simulink model "D53_LKAS_JLU_20200911_1116"  (R2018b)
settings: Solver=ode3  StartTime=0.0  StopTime=10.0  FixedStep=0.01  RelTol=1e-3  EnableMultiTasking=on
model workspace (MAT data in the model file):
  MCOS : class17 (value not decoded)
  MCOS : class17 (value not decoded)
  MCOS : class17 (value not decoded)
  MCOS : class17 (value not decoded)
  MCOS : class17 (value not decoded)
  MCOS : class17 (value not decoded)
  MCOS : class17 (value not decoded)
  MCOS : class17 (value not decoded)
  MCOS : class17 (value not decoded)
  MCOS : class17 (value not decoded)
  MCOS : class17 (value not decoded)
  MCOS : class17 (value not decoded)
  MCOS : class17 (value not decoded)
  MCOS : class17 (value not decoded)
  MCOS : class17 (value not decoded)
  MCOS : class17 (value not decoded)
  MCOS : class17 (value not decoded)
  MCOS : class17 (value not decoded)
  MCOS : class17 (value not decoded)
  MCOS : class17 (value not decoded)
  MCOS : class17 (value not decoded)
  MCOS : class17 (value not decoded)
  MCOS : class17 (value not decoded)
  MCOS : class17 (value not decoded)
  MCOS : class17 (value not decoded)
  MCOS : class17 (value not decoded)
  MCOS : class17 (value not decoded)
  MCOS : class17 (value not decoded)
  MCOS : class17 (value not decoded)
  MCOS : class17 (value not decoded)
  MCOS : class17 (value not decoded)
  MCOS : class17 (value not decoded)
  MCOS : class17 (value not decoded)
  MCOS : class17 (value not decoded)
  MCOS : class17 (value not decoded)
  MCOS : class17 (value not decoded)
  MCOS : class17 (value not decoded)
  MCOS : class17 (value not decoded)
  MCOS : class17 (value not decoded)
  MCOS : class17 (value not decoded)
  MCOS : class17 (value not decoded)
  MCOS : class17 (value not decoded)
  MCOS : class17 (value not decoded)
  MCOS : class17 (value not decoded)
  MCOS : class17 (value not decoded)
  MCOS : class17 (value not decoded)
  MCOS : class17 (value not decoded)
  MCOS : class17 (value not decoded)
  MCOS : class17 (value not decoded)
  MCOS : class17 (value not decoded)
  MCOS : class17 (value not decoded)
  MCOS : class17 (value not decoded)
  MCOS : class17 (value not decoded)
  MCOS : class17 (value not decoded)
  MCOS : class17 (value not decoded)
  MCOS : class17 (value not decoded)
  MCOS : class17 (value not decoded)
  MCOS : class17 (value not decoded)
  MCOS : class17 (value not decoded)
  MCOS : class17 (value not decoded)
  MCOS : class17 (value not decoded)
  MCOS : class17 (value not decoded)
  MCOS : class17 (value not decoded)
  MCOS : class17 (value not decoded)
  MCOS : class17 (value not decoded)
  MCOS : class17 (value not decoded)
  MCOS : class17 (value not decoded)
  MCOS : class17 (value not decoded)
  MCOS : class17 (value not decoded)
  MCOS : class17 (value not decoded)
  MCOS : class17 (value not decoded)
  MCOS : class17 (value not decoded)
  MCOS : class17 (value not decoded)
  MCOS : class17 (value not decoded)
  MCOS : class17 (value not decoded)
  MCOS : class17 (value not decoded)
  MCOS : class17 (value not decoded)
  MCOS : class17 (value not decoded)
  MCOS : class17 (value not decoded)
  MCOS : class17 (value not decoded)
  MCOS : class17 (value not decoded)
  MCOS : class17 (value not decoded)
  MCOS : class17 (value not decoded)
  MCOS : class17 (value not decoded)
  MCOS : class17 (value not decoded)
  MCOS : class17 (value not decoded)
  MCOS : class17 (value not decoded)
  MCOS : class17 (value not decoded)
  MCOS : class17 (value not decoded)
undefined symbols (not defined in the file): LKA_CarWidth, LKA_SampleTime, LKA_StrRatio_C, LKA_Veh2CamL_C, LKA_Veh2CamW_C, LKA_WhlBaseL_C, LL_CompSWA_C, LL_CrvtPrvwT_C, LL_DesDvt_C, LL_DvtComp_C, LL_DvtPrvwT_C, LL_DvtSpdDet_vDvtSpdMin_C, LL_HdAgExT_C, LL_HdAgPrvwT_C, LL_LAccMax_C, LL_LAccRMax_C, LL_LDW_EarliestWarnLine_C, LL_LDW_LatestWarnLine_C, LL_LDWS_SUPPRESS_HEADING, LL_LFClb_TFC_DiffCtlBalance, LL_LFClb_TFC_DiffCtrlMaxSWA, LL_LFClb_TFC_DiffCtrlRatio, LL_LFClb_TFC_facmGainLutGain1_C, LL_LFClb_TFC_facmGainLutGain2_C, LL_LFClb_TFC_facmIntegRatio, LL_LFClb_TFC_facmKlat_C, LL_LFClb_TFC_FfCtlRatio_C, LL_LFClb_TFC_phiIntegCtlMaxSWA_C, LL_LFClb_TFC_tiKlatPrvwT_C, LL_LFClb_TFC_vGainLutVehSpdLwr_C, LL_LFClb_TFC_vGainLutVehSpdUpr_C, LL_LKA_EarliestWarnLine_C, LL_LKA_LatestWarnLine_C, LL_LKAExPrcs_ExitC0Dvt, LL_LKAExPrcs_ExitC0Swt, LL_LKAExPrcs_tiExitTime1, LL_LKAExPrcs_tiExitTime2, LL_LKAExPrcs_tiExitTime3, LL_LKAS_OUT_OF_CONTROL_LAT_VEL, LL_LKAS_OUT_OF_CONTROL_TTLC, LL_LKASWASyn_M0, LL_LKASWASyn_M1, LL_LKASWASyn_M2, LL_LKASWASyn_M3K, LL_LKASWASyn_SWAaddMax, LL_LKASWASyn_T2, LL_LKASWASyn_tiTrqSwaRtTime, LL_LKASWASyn_tiTrqSwaTime, LL_LKASWASyn_TrqMax, LL_LKASWASyn_TrqSwaAddSwt, LL_LKASWASyn_TrqSwaRateDiff, LL_LSpdCompT_C, LL_lStpLngth_C, LL_MAX_DELAY_EPSSTAR_TIME, LL_MAX_DRIVER_TORQUE_DISABLE, LL_MAX_DRIVER_TORQUE_ENABLE, LL_MAX_LANE_WIDTH_DISABLE, LL_MAX_LANE_WIDTH_ENABLE, LL_MAX_LAT_ACC_DISABLE, LL_MAX_LAT_ACC_ENABLE ... (+30)
libraries: simulink x134, canmsglib x52, dspstat3 x3, simulink_extras x1
(part 15 of 18)

== system D53_LKAS_JLU_20200911_1116/LL/LLOn/LL State Determination (LLStateDet)/LL State Machine Conditions (LLSMCon)/Deactivation Condition (DeactvC)/Deviation Threshold Condition (DvtThresCon)/Active Lane Calculation (ActLanCalc) ==
  ActLanCalc_bsL0Info : Inport
  ActLanCalc_bsR0Info : Inport  Port=2
  ActLanCalc_ActvCClb : Inport  Port=3
  Abs2 : Abs
  Abs3 : Abs
  Add1 : Sum
  Add2 : Sum  Inputs=+-
  Bus Creator : BusCreator  Inputs=7
  Bus Selector1 : BusSelector  OutputSignals=R0_C0
  Bus Selector2 : BusSelector  OutputSignals=L0_C0
  Bus Selector3 : BusSelector  OutputSignals=LL_ThresDet_lDvtThresLwrLDW,LL_ThresDet_lDvtThresUprLDW,LL_ThresDet_tiTTLCThresLDW,LL_ThresDet_lDvtThresLwrLKA,LL_ThresDet_lDvtThresUprLKA,LL_ThresDet_tiTTLCThresLKA,LL_DvtSpdDet_vDvtSpdMin_C
  Constant1 : Constant  Value=0.6  OutDataTypeStr=single
  Constant2 : Constant  Value=0.3  OutDataTypeStr=single
  Divide : Product  Inputs=*/
  Divide{1..6} (6 alike) : Product  Inputs=**
  Gain : Gain  Gain=0.25
  Saturation1 : Saturate  UpperLimit=5.5  LowerLimit=2.4
  Saturation2 : Saturate  UpperLimit=0.3  LowerLimit=0
  ActLanCalc_ActvCClbOut : Outport
  wires:
  ActLanCalc_bsL0Info/1 -> Bus Selector2/1
  ActLanCalc_bsR0Info/1 -> Bus Selector1/1
  Bus Selector2/1 -> Abs2/1  "<L0_C0>"
  Bus Selector1/1 -> Abs3/1  "<R0_C0>"
  ActLanCalc_ActvCClb/1 -> Bus Selector3/1
  Gain/1 -> Add2/1
  Add1/1 -> Saturation1/1
  Abs3/1 -> Add1/2
  Constant1/1 -> Add2/2
  Saturation1/1 -> Gain/1
  Abs2/1 -> Add1/1
  Add2/1 -> Saturation2/1
  Bus Selector3/1 -> Divide1/2  "<LL_ThresDet_lDvtThresLwrLDW>"
  Bus Selector3/2 -> Divide2/2  "<LL_ThresDet_lDvtThresUprLDW>"
  Constant2/1 -> Divide/2
  Saturation2/1 -> Divide/1
  Bus Selector3/3 -> Divide3/2  "<LL_ThresDet_tiTTLCThresLDW>"
  Bus Selector3/4 -> Divide4/2  "<LL_ThresDet_lDvtThresLwrLKA>"
  Bus Selector3/5 -> Divide5/2  "<LL_ThresDet_lDvtThresUprLKA>"
  Bus Selector3/6 -> Divide6/2  "<LL_ThresDet_tiTTLCThresLKA>"
  Divide/1 -> Divide2/1, Divide5/1, Divide6/1, Divide4/1, Divide3/1, Divide1/1
  Divide1/1 -> Bus Creator/1  "LL_ThresDet_lDvtThresLwrLDW"
  Divide2/1 -> Bus Creator/2  "LL_ThresDet_lDvtThresUprLDW"
  Divide3/1 -> Bus Creator/3  "LL_ThresDet_tiTTLCThresLDW"
  Divide4/1 -> Bus Creator/4  "LL_ThresDet_lDvtThresLwrLKA"
  Divide5/1 -> Bus Creator/5  "LL_ThresDet_lDvtThresUprLKA"
  Divide6/1 -> Bus Creator/6  "LL_ThresDet_tiTTLCThresLKA"
  Bus Creator/1 -> ActLanCalc_ActvCClbOut/1
  Bus Selector3/7 -> Bus Creator/7  "<LL_DvtSpdDet_vDvtSpdMin_C>"

== system D53_LKAS_JLU_20200911_1116/LL/LLOn/LL State Determination (LLStateDet)/LL State Machine Conditions (LLSMCon)/Deactivation Condition (DeactvC)/Deviation Threshold Condition (DvtThresCon)/Deviation Calculation (DvtCalc) ==
  DvtCalc_bsL0Info : Inport
  DvtCalc_bsR0Info : Inport  Port=2
  Bus Selector1 : BusSelector  OutputSignals=R0_C0,R0_C1
  Bus Selector2 : BusSelector  OutputSignals=L0_C0,L0_C1
  Bus Selector3 : BusSelector  OutputSignals=EnaCClb.LL_DvtComp_C
  Left Front Conner Deviation Calculation (LFCDvtCalc) : Subsystem
  Right Front Conner Deviation Calculation (RFCDvtCalc) : Subsystem
  Saturation : Saturate  UpperLimit=3  LowerLimit=-3
  Saturation1 : Saturate  UpperLimit=0.2  LowerLimit=-0.2
  Saturation2 : Saturate  UpperLimit=3  LowerLimit=-3
  Saturation3 : Saturate  UpperLimit=0.2  LowerLimit=-0.2
  Saturation4 : Saturate  UpperLimit=0.1  LowerLimit=-0.1
  DvtCalc_lLftDvt : Outport
  DvtCalc_lRgtDvt : Outport  Port=2
  wires:
  Saturation4/1 -> Left Front Conner Deviation Calculation (LFCDvtCalc)/3(LFCDvtCalc_lDvtComp_C), Right Front Conner Deviation Calculation (RFCDvtCalc)/3(RFCDvtCalc_lDvtComp)
  Saturation3/1 -> Right Front Conner Deviation Calculation (RFCDvtCalc)/2(RFCDvtCalc_phiHdAg)
  Saturation2/1 -> Right Front Conner Deviation Calculation (RFCDvtCalc)/1(RFCDvtCalc_lDvt)
  Saturation1/1 -> Left Front Conner Deviation Calculation (LFCDvtCalc)/2(LFCDvtCalc_phiHdAg)
  Saturation/1 -> Left Front Conner Deviation Calculation (LFCDvtCalc)/1(LFCDvtCalc_lDvt)
  [LLClb_bsLLSMConClb] -> Bus Selector3/1
  Bus Selector3/1 -> Saturation4/1  "<LL_DvtComp_C>"
  Bus Selector1/2 -> Saturation3/1  "<R0_C1>"
  Bus Selector1/1 -> Saturation2/1  "<R0_C0>"
  Bus Selector2/2 -> Saturation1/1  "<L0_C1>"
  Bus Selector2/1 -> Saturation/1  "<L0_C0>"
  Right Front Conner Deviation Calculation (RFCDvtCalc)/1(DvtCalc_lRgtDvt) -> DvtCalc_lRgtDvt/1
  Left Front Conner Deviation Calculation (LFCDvtCalc)/1(DvtCalc_lLftDvt) -> DvtCalc_lLftDvt/1
  DvtCalc_bsR0Info/1 -> Bus Selector1/1
  DvtCalc_bsL0Info/1 -> Bus Selector2/1

== system D53_LKAS_JLU_20200911_1116/LL/LLOn/LL State Determination (LLStateDet)/LL State Machine Conditions (LLSMCon)/Deactivation Condition (DeactvC)/Deviation Threshold Condition (DvtThresCon)/Deviation Speed Calculation (DvtSpdCalc) ==
  DvtSpdCalc_phiPrvwHdAgLft : Inport
  DvtSpdCalc_phiPrvwHdAgRgt : Inport  Port=2
  DvtSpdCalc_vVehSpd : Inport  Port=3
  Divide : Product  Inputs=**  OutDataTypeStr=single
  Divide1 : Product  Inputs=**  OutDataTypeStr=single
  Gain : Gain  Gain=1/3.6  OutDataTypeStr=single
  DvtSpdCalc_vLftDvtSpd : Outport
  DvtSpdCalc_vRgtDvtSpd : Outport  Port=2
  wires:
  DvtSpdCalc_phiPrvwHdAgLft/1 -> Divide/1
  DvtSpdCalc_phiPrvwHdAgRgt/1 -> Divide1/2
  Gain/1 -> Divide1/1, Divide/2
  DvtSpdCalc_vVehSpd/1 -> Gain/1
  Divide1/1 -> DvtSpdCalc_vRgtDvtSpd/1
  Divide/1 -> DvtSpdCalc_vLftDvtSpd/1

== system D53_LKAS_JLU_20200911_1116/LL/LLOn/LL State Determination (LLStateDet)/LL State Machine Conditions (LLSMCon)/Deactivation Condition (DeactvC)/Deviation Threshold Condition (DvtThresCon)/Deviation Threshold Judgement LDW (DvtThresJdg) ==
  DvtThresJdg_lLftDvt : Inport
  DvtThresJdg_lRgtDvt : Inport  Port=2
  DvtThresJdg_vLftDvtSpd : Inport  Port=3
  DvtThresJdg_vRgtDvtSpd : Inport  Port=4
  DvtThresJdg_tiLftTTLC : Inport  Port=5
  DvtThresJdg_tiRgtTTLC : Inport  Port=6
  DvtThresJdg_bsDvtThresClb : Inport  Port=7
  Bus Selector : BusSelector  OutputSignals=LL_DvtSpdDet_vDvtSpdMin_C
  Deviation Speed Detection (DvtSpdDet) : Subsystem
  Deviation Threshold Condition Synthesis (DTCSyn) : Subsystem
  Left Side Deviation Threshold Condition (LftDTC) : Subsystem
  Right Side Deviation Threshold Condition (RgtDTC) : Subsystem
  DvtThresJdg_stDvtThresActvFlg : Outport
  wires:
  DvtThresJdg_bsDvtThresClb/1 -> Right Side Deviation Threshold Condition (RgtDTC)/1(RgtDTC_bsDvtThresInfo), Left Side Deviation Threshold Condition (LftDTC)/1(LftDTC_bsDvtThresInfo), Bus Selector/1
  DvtThresJdg_lLftDvt/1 -> Left Side Deviation Threshold Condition (LftDTC)/2(LftDTC_lLftDvt)
  DvtThresJdg_vLftDvtSpd/1 -> Deviation Speed Detection (DvtSpdDet)/1(DvtSpdDet_vLftDvtSpd), Left Side Deviation Threshold Condition (LftDTC)/3(LftDTC_vLftDvtSpd)
  DvtThresJdg_tiLftTTLC/1 -> Left Side Deviation Threshold Condition (LftDTC)/4(LftDTC_tiLftTTLC)
  DvtThresJdg_tiRgtTTLC/1 -> Right Side Deviation Threshold Condition (RgtDTC)/4(RgtDTC_tiRgtTTLC)
  DvtThresJdg_lRgtDvt/1 -> Right Side Deviation Threshold Condition (RgtDTC)/2(RgtDTC_lRgtDvt)
  DvtThresJdg_vRgtDvtSpd/1 -> Deviation Speed Detection (DvtSpdDet)/2(DvtSpdDet_vRgtDvtSpd), Right Side Deviation Threshold Condition (RgtDTC)/3(RgtDTC_vRgtDvtSpd)
  Left Side Deviation Threshold Condition (LftDTC)/1(LftDTC_stLftDvtThresActvFlg) -> Deviation Threshold Condition Synthesis (DTCSyn)/1(DTCSyn_stLftDvtThresActvFlg)
  Right Side Deviation Threshold Condition (RgtDTC)/1(RgtDTC_stRgtDvtThresActvFlg) -> Deviation Threshold Condition Synthesis (DTCSyn)/2(DTCSyn_stRgtDvtThresActvFlg)
  Deviation Threshold Condition Synthesis (DTCSyn)/1(DTCSyn_stDvtThresActvFlg) -> DvtThresJdg_stDvtThresActvFlg/1
  Deviation Speed Detection (DvtSpdDet)/1(DvtSpdDet_stDvtSpdFlg) -> Deviation Threshold Condition Synthesis (DTCSyn)/3(DTCSyn_stDvtSpdFlg)
  Bus Selector/1 -> Deviation Speed Detection (DvtSpdDet)/3(DvtSpdDet_vDvtSpdMin_C)  "<LL_DvtSpdDet_vDvtSpdMin_C>"

== system D53_LKAS_JLU_20200911_1116/LL/LLOn/LL State Determination (LLStateDet)/LL State Machine Conditions (LLSMCon)/Deactivation Condition (DeactvC)/Deviation Threshold Condition (DvtThresCon)/Deviation Threshold Judgement LKA (DvtThresJdg) ==
  DvtThresJdg_lLftDvt : Inport
  DvtThresJdg_lRgtDvt : Inport  Port=2
  DvtThresJdg_vLftDvtSpd : Inport  Port=3
  DvtThresJdg_vRgtDvtSpd : Inport  Port=4
  DvtThresJdg_tiLftTTLC : Inport  Port=5
  DvtThresJdg_tiRgtTTLC : Inport  Port=6
  DvtThresJdg_bsDvtThresClb : Inport  Port=7
  Bus Selector : BusSelector  OutputSignals=LL_DvtSpdDet_vDvtSpdMin_C
  Deviation Speed Detection (DvtSpdDet) : Subsystem
  Deviation Threshold Condition Synthesis (DTCSyn) : Subsystem
  Left Side Deviation Threshold Condition (LftDTC) : Subsystem
  Right Side Deviation Threshold Condition (RgtDTC) : Subsystem
  DvtThresJdg_stDvtThresActvFlg : Outport
  wires:
  Bus Selector/1 -> Deviation Speed Detection (DvtSpdDet)/3(DvtSpdDet_vDvtSpdMin_C)  "<LL_DvtSpdDet_vDvtSpdMin_C>"
  Deviation Speed Detection (DvtSpdDet)/1(DvtSpdDet_stDvtSpdFlg) -> Deviation Threshold Condition Synthesis (DTCSyn)/3(DTCSyn_stDvtSpdFlg)
  Deviation Threshold Condition Synthesis (DTCSyn)/1(DTCSyn_stDvtThresActvFlg) -> DvtThresJdg_stDvtThresActvFlg/1
  Right Side Deviation Threshold Condition (RgtDTC)/1(RgtDTC_stRgtDvtThresActvFlg) -> Deviation Threshold Condition Synthesis (DTCSyn)/2(DTCSyn_stRgtDvtThresActvFlg)
  Left Side Deviation Threshold Condition (LftDTC)/1(LftDTC_stLftDvtThresActvFlg) -> Deviation Threshold Condition Synthesis (DTCSyn)/1(DTCSyn_stLftDvtThresActvFlg)
  DvtThresJdg_vRgtDvtSpd/1 -> Right Side Deviation Threshold Condition (RgtDTC)/3(RgtDTC_vRgtDvtSpd), Deviation Speed Detection (DvtSpdDet)/2(DvtSpdDet_vRgtDvtSpd)
  DvtThresJdg_lRgtDvt/1 -> Right Side Deviation Threshold Condition (RgtDTC)/2(RgtDTC_lRgtDvt)
  DvtThresJdg_tiRgtTTLC/1 -> Right Side Deviation Threshold Condition (RgtDTC)/4(RgtDTC_tiRgtTTLC)
  DvtThresJdg_tiLftTTLC/1 -> Left Side Deviation Threshold Condition (LftDTC)/4(LftDTC_tiLftTTLC)
  DvtThresJdg_vLftDvtSpd/1 -> Left Side Deviation Threshold Condition (LftDTC)/3(LftDTC_vLftDvtSpd), Deviation Speed Detection (DvtSpdDet)/1(DvtSpdDet_vLftDvtSpd)
  DvtThresJdg_lLftDvt/1 -> Left Side Deviation Threshold Condition (LftDTC)/2(LftDTC_lLftDvt)
  DvtThresJdg_bsDvtThresClb/1 -> Bus Selector/1, Left Side Deviation Threshold Condition (LftDTC)/1(LftDTC_bsDvtThresInfo), Right Side Deviation Threshold Condition (RgtDTC)/1(RgtDTC_bsDvtThresInfo)

== system D53_LKAS_JLU_20200911_1116/LL/LLOn/LL State Determination (LLStateDet)/LL State Machine Conditions (LLSMCon)/Deactivation Condition (DeactvC)/Driver Take Condition (DvrTkCon)/Count ==
  Input : Inport
  Enable : EnablePort  StatesWhenEnabling=reset
  Add : Sum
  Cast To Single : DataTypeConversion  OutDataTypeStr=uint16
  Memory : Memory  InheritSampleTime=on
  Saturation : Saturate  UpperLimit=50000  LowerLimit=0
  Out : Outport  OutputWhenDisabled=reset  InitialOutput=0
  wires:
  Memory/1 -> Add/2
  Add/1 -> Saturation/1
  Input/1 -> Cast To Single/1
  Saturation/1 -> Out/1, Memory/1
  Cast To Single/1 -> Add/1

== system D53_LKAS_JLU_20200911_1116/LL/LLOn/LL State Determination (LLStateDet)/LL State Machine Conditions (LLSMCon)/Deactivation Condition (DeactvC)/Driver Take Condition (DvrTkCon)/Count 0.2s ==
  Input : Inport
  Input1 : Inport  Port=2
  Enable : EnablePort  StatesWhenEnabling=reset
  Add : Sum
  Cast To Single : DataTypeConversion  OutDataTypeStr=uint16
  Memory : Memory  InheritSampleTime=on
  Relational Operator : RelationalOperator  OutDataTypeStr=boolean  RndMeth=Nearest
  Saturation : Saturate  UpperLimit=50000  LowerLimit=0
  Out : Outport  OutputWhenDisabled=reset  InitialOutput=0
  wires:
  Input1/1 -> Relational Operator/2
  Cast To Single/1 -> Add/1
  Relational Operator/1 -> Out/1
  Input/1 -> Cast To Single/1
  Add/1 -> Saturation/1
  Saturation/1 -> Memory/1, Relational Operator/1
  Memory/1 -> Add/2

== system D53_LKAS_JLU_20200911_1116/LL/LLOn/LL State Determination (LLStateDet)/LL State Machine Conditions (LLSMCon)/Deactivation Condition (DeactvC)/Driver Take Condition (DvrTkCon)/Time Delay (TDel) ==
  TDel_stFlgIn : Inport
  TDel_tiTDel : Inport  Port=2
  Detect Fall Nonpositive : simulink/Logic and Bit Operations/Detect Fall Nonpositive  vinit=0  OutDataTypeStr=boolean
      settings: SourceProductName=Simulink  SourceProductBaseCode=SL
  Detect Rise Positive : simulink/Logic and Bit Operations/Detect Rise Positive  vinit=0  OutDataTypeStr=boolean
  If : If  NumInputs=4  IfExpression=u1 & u2  ElseIfExpressions=(~u3) & u4
  If Action Subsystem : Subsystem  TreatAsAtomicUnit=on
  If Action Subsystem1 : Subsystem  TreatAsAtomicUnit=on
  If Action Subsystem3 : Subsystem  TreatAsAtomicUnit=on
  Merge : Merge  Inputs=3
  Sum Condition1 : Subsystem  TreatAsAtomicUnit=on
  Unit Delay : UnitDelay  SampleTime=-1
  TDel_stFlgOut : Outport
  wires:
  TDel_tiTDel/1 -> Sum Condition1/2(Sum)
  Detect Fall Nonpositive/1 -> If/4
  Detect Rise Positive/1 -> If/2
  TDel_stFlgIn/1 -> If/1, Detect Rise Positive/1
  Sum Condition1/1(Out) -> Unit Delay/1, TDel_stFlgOut/1
  Unit Delay/1 -> If/3, Detect Fall Nonpositive/1, If Action Subsystem3/1(In1)
  Merge/1 -> Sum Condition1/Enable, Sum Condition1/1(In)
  If Action Subsystem3/1(Out) -> Merge/3
  If Action Subsystem1/1(Out) -> Merge/2
  If Action Subsystem/1(Out) -> Merge/1
  If/3 -> If Action Subsystem3/Action
  If/2 -> If Action Subsystem1/Action
  If/1 -> If Action Subsystem/Action

== system D53_LKAS_JLU_20200911_1116/LL/LLOn/LL State Determination (LLStateDet)/LL State Machine Conditions (LLSMCon)/Deactivation Condition (DeactvC)/EPS Condition (EPSC)/Sum Condition1 ==
  In : Inport
  Sum : Inport  Port=2
  state = reset : EnablePort  StatesWhenEnabling=reset
  Add1 : Sum  OutDataTypeStr=uint16
  Data Type Conversion : DataTypeConversion  OutDataTypeStr=boolean
  Memory : Memory  InheritSampleTime=on
  Relational Operator : RelationalOperator  OutDataTypeStr=boolean  RndMeth=Nearest
  Saturation : Saturate  UpperLimit=100  LowerLimit=0
  Out : Outport  OutputWhenDisabled=reset  InitialOutput=0
  wires:
  Saturation/1 -> Relational Operator/1, Memory/1
  Data Type Conversion/1 -> Out/1
  Sum/1 -> Relational Operator/2
  In/1 -> Add1/1
  Add1/1 -> Saturation/1
  Memory/1 -> Add1/2
  Relational Operator/1 -> Data Type Conversion/1

== system D53_LKAS_JLU_20200911_1116/LL/LLOn/LL State Determination (LLStateDet)/LL State Machine Conditions (LLSMCon)/Disable Condition (DisblC)/Disable Condition Synthesis (DisblCSyn)/If Action Subsystem1 ==
  Action Port : ActionPort  InitializeStates=reset  ActionType=then
  Constant : Constant  OutDataTypeStr=boolean  SampleTime=-1
  Out : Outport  InitialOutput=1
  wires:
  Constant/1 -> Out/1

== system D53_LKAS_JLU_20200911_1116/LL/LLOn/LL State Determination (LLStateDet)/LL State Machine Conditions (LLSMCon)/Disable Condition (DisblC)/Disable Condition Synthesis (DisblCSyn)/If Action Subsystem2 ==
  Action Port : ActionPort  InitializeStates=reset  ActionType=then
  Constant : Constant  OutDataTypeStr=boolean  SampleTime=-1
  Out : Outport  InitialOutput=1
  wires:
  Constant/1 -> Out/1

== system D53_LKAS_JLU_20200911_1116/LL/LLOn/LL State Determination (LLStateDet)/LL State Machine Conditions (LLSMCon)/Disable Condition (DisblC)/Disable Condition Synthesis (DisblCSyn)/If Action Subsystem3 ==
  Action Port : ActionPort  InitializeStates=reset  ActionType=else
  Constant : Constant  Value=0  OutDataTypeStr=boolean
  Out : Outport  InitialOutput=0
  wires:
  Constant/1 -> Out/1

== system D53_LKAS_JLU_20200911_1116/LL/LLOn/LL State Determination (LLStateDet)/LL State Machine Conditions (LLSMCon)/Disable Condition (DisblC)/Disable Condition Synthesis (DisblCSyn)/If Action Subsystem4 ==
  Action Port : ActionPort  InitializeStates=reset  ActionType=else
  Constant : Constant  Value=0  OutDataTypeStr=boolean
  Out : Outport  InitialOutput=0
  wires:
  Constant/1 -> Out/1

== system D53_LKAS_JLU_20200911_1116/LL/LLOn/LL State Determination (LLStateDet)/LL State Machine Conditions (LLSMCon)/Disable Condition (DisblC)/Driver Intent Condition (DrvInttC)/Driver Action Condition Synthesis (DrvActnCSyn) ==
  DrvActnCSyn_stTkOvStActvFlg : Inport
  DrvActnCSyn_stDrvRlsDetFlg : Inport  Port=2
  DrvActnCSyn_stTkOvStChk : Inport  Port=3
  Logical Operator1 : Logic  Operator=OR  Inputs=3  AllPortsSameDT=off  OutDataTypeStr=boolean
  DrvActnCSyn_stDrvActnCSyn : Outport
  wires:
  DrvActnCSyn_stDrvRlsDetFlg/1 -> Logical Operator1/2
  DrvActnCSyn_stTkOvStActvFlg/1 -> Logical Operator1/1
  DrvActnCSyn_stTkOvStChk/1 -> Logical Operator1/3
  Logical Operator1/1 -> DrvActnCSyn_stDrvActnCSyn/1

== system D53_LKAS_JLU_20200911_1116/LL/LLOn/LL State Determination (LLStateDet)/LL State Machine Conditions (LLSMCon)/Disable Condition (DisblC)/Driver Intent Condition (DrvInttC)/Driver Action Detection (DrvActnDet) ==
  DrvActnDet_phiSWA : Inport
  DrvActnDet_aLAcc : Inport  Port=2
  DrvActnDet_aFAcc : Inport  Port=3
  DrvActnDet_phiSWAMax_C : Inport  Port=4
  DrvActnDet_dphiSWARateMax_C : Inport  Port=5
  DrvActnDet_aLAccMax_C : Inport  Port=6
  DrvActnDet_aFAccMax_C : Inport  Port=7
  DrvActnDet_aFAccMin_C : Inport  Port=8
  DrvActnDet_bsEPSInfo : Inport  Port=9
  Abs2 : Abs  OutDataTypeStr=single
  Abs3 : Abs  OutDataTypeStr=single
  Abs4 : Abs  OutDataTypeStr=single
  Bus Creator : BusCreator  Inputs=4
  Bus Selector : BusSelector  OutputSignals=EPS_LKA_State
  Compare To Constant : simulink/Logic and Bit Operations/Compare To Constant  relop=~=  const=3.0  OutDataTypeStr=boolean
  Compare To Constant2 : simulink/Logic and Bit Operations/Compare To Constant  relop===  const=0  OutDataTypeStr=boolean
  Discrete Derivative : simulink/Discrete/Discrete Derivative  gainval=1.0  ICPrevScaledInput=0.0  OutMin=[]  OutMax=[]  OutDataTypeStr=single  OutputDataTypeScalingMode=single  OutDataType=fixdt(1, 16)  OutScaling=2^-10  DoSatur=off
  Interval Test Dynamic : simulink/Logic and Bit Operations/Interval Test Dynamic  IntervalClosedRight=off  IntervalClosedLeft=off  OutDataTypeStr=boolean
      settings: SourceProductName=Simulink  SourceProductBaseCode=SL
  Logical Operator : Logic  Operator=OR  Inputs=4  AllPortsSameDT=off  OutDataTypeStr=boolean
  Logical Operator1 : Logic  AllPortsSameDT=off  OutDataTypeStr=boolean
  Relational Operator1 : RelationalOperator  OutDataTypeStr=boolean  RndMeth=Nearest
  Relational Operator2 : RelationalOperator  OutDataTypeStr=boolean  RndMeth=Nearest
  Relational Operator3 : RelationalOperator  OutDataTypeStr=boolean  RndMeth=Nearest
  Unary Minus : UnaryMinus
  DrvActnDet_stTkOvStActvFlg : Outport
  DrvActnDet : Outport  Port=2
  wires:
  Relational Operator2/1 -> Logical Operator/2, Bus Creator/2  "dphiSWARate_Thres"
  Logical Operator1/1 -> Logical Operator/3, Bus Creator/3  "aLAcc_Thres"
  Compare To Constant2/1 -> Logical Operator/4, Bus Creator/4  "aFLAcc_Thres"
  Bus Creator/1 -> DrvActnDet/1
  Relational Operator1/1 -> Logical Operator/1, Bus Creator/1  "phiSWA_Thres"
  Logical Operator/1 -> DrvActnDet_stTkOvStActvFlg/1
  Compare To Constant/1 -> Logical Operator1/2
  Bus Selector/1 -> Compare To Constant/1  "<EPS_LKA_State>"
  DrvActnDet_bsEPSInfo/1 -> Bus Selector/1
  Relational Operator3/1 -> Logical Operator1/1
  Unary Minus/1 -> Interval Test Dynamic/3
  DrvActnDet_aFAccMax_C/1 -> Interval Test Dynamic/1
  Interval Test Dynamic/1 -> Compare To Constant2/1
  DrvActnDet_aFAcc/1 -> Interval Test Dynamic/2
  DrvActnDet_aFAccMin_C/1 -> Unary Minus/1
  DrvActnDet_aLAccMax_C/1 -> Relational Operator3/2
  Abs4/1 -> Relational Operator3/1
  DrvActnDet_aLAcc/1 -> Abs4/1
  Discrete Derivative/1 -> Abs3/1
  DrvActnDet_dphiSWARateMax_C/1 -> Relational Operator2/2
  Abs3/1 -> Relational Operator2/1
  DrvActnDet_phiSWAMax_C/1 -> Relational Operator1/2
  Abs2/1 -> Relational Operator1/1
  DrvActnDet_phiSWA/1 -> Abs2/1, Discrete Derivative/1

== system D53_LKAS_JLU_20200911_1116/LL/LLOn/LL State Determination (LLStateDet)/LL State Machine Conditions (LLSMCon)/Disable Condition (DisblC)/Driver Intent Condition (DrvInttC)/Driver Release Detection (DrvRlsDet) ==
  DrvRlsDet_bsEPSInfo : Inport
  Abs : Abs
  Bus Selector1 : BusSelector  OutputSignals=LKA_SampleTime
  Bus Selector2 : BusSelector  OutputSignals=EPS_LKA_State,EPS_SW_Trq
  Cast To Single1 : DataTypeConversion  OutDataTypeStr=uint16
  Compare1 : simulink/Logic and Bit Operations/Compare To Constant  relop===  const=3  OutDataTypeStr=boolean
  Compare3 : simulink/Logic and Bit Operations/Compare To Constant  relop===  const=3  OutDataTypeStr=boolean
  Compare4 : simulink/Logic and Bit Operations/Compare To Constant  relop===  const=1  OutDataTypeStr=boolean
  Constant : Constant  Value=0.25  OutDataTypeStr=single
  Constant1 : Constant  Value=0.5  OutDataTypeStr=single
  Constant2 : Constant  Value=20  OutDataTypeStr=single
  Count 20s : Subsystem
  Divide : Product  Inputs=*/  OutDataTypeStr=single
  Logical Operator1 : Logic  AllPortsSameDT=off  OutDataTypeStr=boolean
  Logical Operator2 : Logic  Operator=OR  AllPortsSameDT=off  OutDataTypeStr=boolean
  Relational Operator : RelationalOperator  Operator=<=  OutDataTypeStr=boolean  RndMeth=Nearest
  Switch : Switch  Criteria=u2 > Threshold
  DrvRlsDet_stDrvRlsDetFlg : Outport
  wires:
  Cast To Single1/1 -> Count 20s/2(Input1)
  Constant2/1 -> Divide/1
  Divide/1 -> Cast To Single1/1
  [LLClb_bsConstantClb] -> Bus Selector1/1
  Bus Selector1/1 -> Divide/2  "<LKA_SampleTime>"
  Abs/1 -> Relational Operator/1
  Count 20s/1(Out) -> DrvRlsDet_stDrvRlsDetFlg/1
  Compare4/1 -> Logical Operator2/1
  Logical Operator1/1 -> Count 20s/1(Input)
  Logical Operator2/1 -> Logical Operator1/1
  Switch/1 -> Relational Operator/2
  Constant1/1 -> Switch/1
  Constant/1 -> Switch/3
  Compare3/1 -> Logical Operator2/2
  Compare1/1 -> Switch/2
  Relational Operator/1 -> Count 20s/Enable, Logical Operator1/2
  Bus Selector2/2 -> Abs/1  "<EPS_SW_Trq>"
  Bus Selector2/1 -> Compare3/1, Compare4/1, Compare1/1  "<EPS_LKA_State>"
  DrvRlsDet_bsEPSInfo/1 -> Bus Selector2/1

== system D53_LKAS_JLU_20200911_1116/LL/LLOn/LL State Determination (LLStateDet)/LL State Machine Conditions (LLSMCon)/Disable Condition (DisblC)/Driver Intent Condition (DrvInttC)/Take-Over Steering Check (TkOvStChk) ==
  TkOvStChk_bsVehSpd : Inport
  TkOvStChk_bsEPSInfo : Inport  Port=2
  TkOvStChk_trqSWTrqMax_C : Inport  Port=3
  TkOvStChk_tiTrqChkT_C : Inport  Port=4
  TkOvStChk_tiTDel_C : Inport  Port=5
  TkOvStChk_crPrvwCrvt : Inport  Port=6
  Abs : Abs
  Abs1 : Abs
  Add : Sum
  Bus Selector : BusSelector  OutputSignals=EPS_SW_Trq
  Bus Selector2 : BusSelector  OutputSignals=LKA_SampleTime
  Cast To Single1 : DataTypeConversion  OutDataTypeStr=uint16
  Cast To Single2 : DataTypeConversion  OutDataTypeStr=uint16
  Cast To Single3 : DataTypeConversion  LockScale=on
  Constant : Constant  Value=0.005  OutDataTypeStr=single
  Divide : Product  Inputs=*/
  Divide1 : Product  Inputs=*/  OutDataTypeStr=single
  Divide2 : Product  Inputs=*/  OutDataTypeStr=single
  Fcn : Fcn  Expr=1.5*u(2)-u(1)/180*u(2)
  Mux : Mux  Inputs=2
  Relational Operator : RelationalOperator  OutDataTypeStr=boolean  RndMeth=Nearest
  Saturation : Saturate  UpperLimit=80  LowerLimit=60
  Saturation1 : Saturate  UpperLimit=2.75  LowerLimit=1.5
  Sum Condition2 : Subsystem  TreatAsAtomicUnit=on
  Time Delay (TDel) : Subsystem
  TkOvStChk_stTkOvStChk : Outport
  wires:
  Saturation1/1 -> Relational Operator/2
  Cast To Single2/1 -> Time Delay (TDel)/2(TDel_tiTDel)
  Cast To Single1/1 -> Sum Condition2/2(Sum)
  Cast To Single3/1 -> Add/2
  Constant/1 -> Divide2/2
  Divide2/1 -> Cast To Single3/1
  Abs1/1 -> Divide2/1
  TkOvStChk_crPrvwCrvt/1 -> Abs1/1
  Add/1 -> Saturation1/1
  Divide1/1 -> Cast To Single2/1
  Divide/1 -> Cast To Single1/1
  [LLClb_bsConstantClb] -> Bus Selector2/1
  Bus Selector2/1 -> Divide/2, Divide1/2  "<LKA_SampleTime>"
  Fcn/1 -> Add/1
  TkOvStChk_tiTDel_C/1 -> Divide1/1
  Sum Condition2/1(Out) -> Time Delay (TDel)/1(TDel_stFlgIn)
  Saturation/1 -> Mux/1
  Mux/1 -> Fcn/1
  TkOvStChk_bsVehSpd/1 -> Saturation/1
  Time Delay (TDel)/1(TDel_stFlgOut) -> TkOvStChk_stTkOvStChk/1
  TkOvStChk_tiTrqChkT_C/1 -> Divide/1
  Relational Operator/1 -> Sum Condition2/Enable, Sum Condition2/1(In)
  TkOvStChk_trqSWTrqMax_C/1 -> Mux/2
  Abs/1 -> Relational Operator/1
  Bus Selector/1 -> Abs/1  "<EPS_SW_Trq>"
  TkOvStChk_bsEPSInfo/1 -> Bus Selector/1

== system D53_LKAS_JLU_20200911_1116/LL/LLOn/LL State Determination (LLStateDet)/LL State Machine Conditions (LLSMCon)/Disable Condition (DisblC)/LDW Alarm Timeout (LDWAlrmTOut)/If Action Subsystem ==
  In : Inport
  Action Port : ActionPort  InitializeStates=reset  ActionType=then
  Add1 : Sum  OutDataTypeStr=single
  Constant1 : Constant  OutDataTypeStr=uint16
  Data Type Conversion : DataTypeConversion  OutDataTypeStr=boolean
  Memory : Memory  InheritSampleTime=on
  Relational Operator : RelationalOperator  OutDataTypeStr=boolean  RndMeth=Nearest
  Saturation : Saturate  UpperLimit=10000  LowerLimit=0
  Out : Outport  InitialOutput=0
  wires:
  Constant1/1 -> Add1/1
  Data Type Conversion/1 -> Out/1
  Add1/1 -> Saturation/1
  Saturation/1 -> Relational Operator/1, Memory/1
  In/1 -> Relational Operator/2
  Memory/1 -> Add1/2
  Relational Operator/1 -> Data Type Conversion/1

== system D53_LKAS_JLU_20200911_1116/LL/LLOn/LL State Determination (LLStateDet)/LL State Machine Conditions (LLSMCon)/Disable Condition (DisblC)/LDW Alarm Timeout (LDWAlrmTOut)/If Action Subsystem1 ==
  Action Port : ActionPort  InitializeStates=reset  ActionType=else
  Constant : Constant  Value=0  OutDataTypeStr=boolean
  Out1 : Outport  InitialOutput=0
  wires:
  Constant/1 -> Out1/1

== system D53_LKAS_JLU_20200911_1116/LL/LLOn/LL State Determination (LLStateDet)/LL State Machine Conditions (LLSMCon)/Disable Condition (DisblC)/LDW Own Condition (LDWOwnC)/LDW Own Condition Synthesis (LDWOwnCSyn) ==
  LDWOwnCSyn_stDACMode : Inport
  LDWOwnCSyn_stVehPosChk : Inport  Port=2
  Compare To Constant : simulink/Logic and Bit Operations/Compare To Constant  relop=>=  const=1  OutDataTypeStr=boolean
  Compare To Constant1 : simulink/Logic and Bit Operations/Compare To Constant  relop===  const=1  OutDataTypeStr=boolean
  Logical Operator : Logic  AllPortsSameDT=off  OutDataTypeStr=boolean
  LDWOwnCSyn_stLDWOwnCSyn : Outport
  wires:
  Logical Operator/1 -> LDWOwnCSyn_stLDWOwnCSyn/1
  Compare To Constant1/1 -> Logical Operator/2
  Compare To Constant/1 -> Logical Operator/1
  LDWOwnCSyn_stVehPosChk/1 -> Compare To Constant1/1
  LDWOwnCSyn_stDACMode/1 -> Compare To Constant/1

== system D53_LKAS_JLU_20200911_1116/LL/LLOn/LL State Determination (LLStateDet)/LL State Machine Conditions (LLSMCon)/Disable Condition (DisblC)/LDW Own Condition (LDWOwnC)/Vehicle Position Check (VehPosChk) ==
  VehPosChk_bsPrDvtInfo : Inport
  VehPosChk_LatestLine_C : Inport  Port=2
  Bus Selector : BusSelector  OutputSignals=ILftDvt,IRgtDvt
  Logical Operator : Logic  Operator=OR  AllPortsSameDT=off  OutDataTypeStr=boolean
  Relational Operator1 : RelationalOperator  Operator=<=  OutDataTypeStr=boolean  RndMeth=Nearest
  Relational Operator2 : RelationalOperator  Operator=<=  OutDataTypeStr=boolean  RndMeth=Nearest
  VehPosChk_stVehPosChk : Outport
  wires:
  Bus Selector/2 -> Relational Operator2/1  "<IRgtDvt>"
  Bus Selector/1 -> Relational Operator1/1  "<ILftDvt>"
  VehPosChk_bsPrDvtInfo/1 -> Bus Selector/1
  Logical Operator/1 -> VehPosChk_stVehPosChk/1
  Relational Operator2/1 -> Logical Operator/2
  Relational Operator1/1 -> Logical Operator/1
  VehPosChk_LatestLine_C/1 -> Relational Operator2/2, Relational Operator1/2

== system D53_LKAS_JLU_20200911_1116/LL/LLOn/LL State Determination (LLStateDet)/LL State Machine Conditions (LLSMCon)/Disable Condition (DisblC)/LKA Own Condition (LKAOwnC)/EPS Condition (EPSC) ==
  EPSC_bsEPSInfo : Inport
  EPSC_bsLLState : Inport  Port=2
  EPSC_tiDelT_C : Inport  Port=3
  Bus Selector : BusSelector  OutputSignals=EPS_LKA_State
  Bus Selector1 : BusSelector  OutputSignals=LKA_State
  Bus Selector2 : BusSelector  OutputSignals=LKA_SampleTime
  Cast To Single1 : DataTypeConversion  OutDataTypeStr=uint16
  Divide : Product  Inputs=*/  OutDataTypeStr=single
  If : If  NumInputs=2  IfExpression=u2 ==3 & u1 ~=1  ElseIfExpressions=(u2 == 4 | u2 == 5)& u1 ~= 3
  If Action Subsystem : Subsystem  TreatAsAtomicUnit=on
  If Action Subsystem1 : Subsystem  TreatAsAtomicUnit=on
  If Action Subsystem3 : Subsystem  TreatAsAtomicUnit=on
  Merge : Merge  Inputs=3
  Sum Condition1 : Subsystem  TreatAsAtomicUnit=on
  EPSC_stEPSC : Outport
  wires:
  Cast To Single1/1 -> Sum Condition1/2(Sum)
  Divide/1 -> Cast To Single1/1
  [LLClb_bsConstantClb] -> Bus Selector2/1
  Bus Selector2/1 -> Divide/2  "<LKA_SampleTime>"
  EPSC_tiDelT_C/1 -> Divide/1
  Bus Selector1/1 -> If/2  "<LKA_State>"
  EPSC_bsLLState/1 -> Bus Selector1/1
  Bus Selector/1 -> If/1  "<EPS_LKA_State>"
  Merge/1 -> Sum Condition1/Enable, Sum Condition1/1(In)
  If Action Subsystem3/1(Out) -> Merge/3
  If/2 -> If Action Subsystem1/Action
  If/3 -> If Action Subsystem3/Action
  If/1 -> If Action Subsystem/Action
  If Action Subsystem/1(Out) -> Merge/1
  If Action Subsystem1/1(Out) -> Merge/2
  Sum Condition1/1(Out) -> EPSC_stEPSC/1
  EPSC_bsEPSInfo/1 -> Bus Selector/1

== system D53_LKAS_JLU_20200911_1116/LL/LLOn/LL State Determination (LLStateDet)/LL State Machine Conditions (LLSMCon)/Disable Condition (DisblC)/LKA Own Condition (LKAOwnC)/LKA Own Condition Synthesis (LKAOwnCSyn) ==
  LKAOwnCSyn_stDACMode : Inport
  LKAOwnCSyn_stVehLSpdC : Inport  Port=2
  LKAOwnCSyn_stVehPosChk : Inport  Port=3
  LKAOwnCSyn_stEPSCtlEC : Inport  Port=4
  Compare To Constant : simulink/Logic and Bit Operations/Compare To Constant  relop===  const=2  OutDataTypeStr=boolean
  Compare To Constant1 : simulink/Logic and Bit Operations/Compare To Constant  relop===  const=1  OutDataTypeStr=boolean
  Compare To Constant2 : simulink/Logic and Bit Operations/Compare To Constant  relop===  const=1  OutDataTypeStr=boolean
  Compare To Constant3 : simulink/Logic and Bit Operations/Compare To Constant  relop===  const=1  OutDataTypeStr=boolean
  Logical Operator : Logic  AllPortsSameDT=off  OutDataTypeStr=boolean
  Logical Operator1 : Logic  Operator=OR  Inputs=3  AllPortsSameDT=off  OutDataTypeStr=boolean
  LKAOwnCSyn_stLKAOwnCSyn : Outport
  wires:
  Compare To Constant3/1 -> Logical Operator1/1
  LKAOwnCSyn_stVehLSpdC/1 -> Compare To Constant3/1
  Logical Operator1/1 -> Logical Operator/2
  Compare To Constant/1 -> Logical Operator/1
  Compare To Constant1/1 -> Logical Operator1/2
  Compare To Constant2/1 -> Logical Operator1/3
  LKAOwnCSyn_stEPSCtlEC/1 -> Compare To Constant2/1
  Logical Operator/1 -> LKAOwnCSyn_stLKAOwnCSyn/1
  LKAOwnCSyn_stVehPosChk/1 -> Compare To Constant1/1
  LKAOwnCSyn_stDACMode/1 -> Compare To Constant/1

== system D53_LKAS_JLU_20200911_1116/LL/LLOn/LL State Determination (LLStateDet)/LL State Machine Conditions (LLSMCon)/Disable Condition (DisblC)/LKA Own Condition (LKAOwnC)/Vehicle Lateral Speed Condition (VehLSpdC) ==
  VehLSpdC_bsTTLC : Inport
  VehLSpdC_vVehLSpdMax_C : Inport  Port=2
  Abs : Abs
  Abs1 : Abs
  Bus Selector : BusSelector  OutputSignals=vLft,vRgt
  Logical Operator : Logic  Operator=OR  AllPortsSameDT=off  OutDataTypeStr=boolean
  Relational Operator1 : RelationalOperator  OutDataTypeStr=boolean  RndMeth=Nearest
  Relational Operator2 : RelationalOperator  OutDataTypeStr=boolean  RndMeth=Nearest
  VehLSpdC_stVehLSpdC : Outport
  wires:
  Logical Operator/1 -> VehLSpdC_stVehLSpdC/1
  Relational Operator2/1 -> Logical Operator/2
  Relational Operator1/1 -> Logical Operator/1
  VehLSpdC_vVehLSpdMax_C/1 -> Relational Operator1/2, Relational Operator2/2
  Abs1/1 -> Relational Operator2/1
  Bus Selector/2 -> Abs1/1  "<vRgt>"
  Bus Selector/1 -> Abs/1  "<vLft>"
  Abs/1 -> Relational Operator1/1
  VehLSpdC_bsTTLC/1 -> Bus Selector/1

== system D53_LKAS_JLU_20200911_1116/LL/LLOn/LL State Determination (LLStateDet)/LL State Machine Conditions (LLSMCon)/Disable Condition (DisblC)/LKA Own Condition (LKAOwnC)/Vehicle Position Check (VehPosChk) ==
  VehPosChk_bsL0Info : Inport
  VehPosChk_bsR0Info : Inport  Port=2
  VehPosChk_DvtComp_C : Inport  Port=3
  VehPosChk_lAlrmLine_C : Inport  Port=4
  Bus Selector : BusSelector  OutputSignals=L0_C0
  Bus Selector1 : BusSelector  OutputSignals=R0_C0
  Left Front Conner Deviation Calculation (LFCDvtCalc) : Subsystem
  Logical Operator : Logic  Operator=OR  AllPortsSameDT=off  OutDataTypeStr=boolean
  Relational Operator1 : RelationalOperator  Operator=<=  OutDataTypeStr=boolean  RndMeth=Nearest
  Relational Operator2 : RelationalOperator  Operator=<=  OutDataTypeStr=boolean  RndMeth=Nearest
  Right Front Conner Deviation Calculation (RFCDvtCalc) : Subsystem
  VehPosChk_stVehPosChk : Outport
  wires:
  Logical Operator/1 -> VehPosChk_stVehPosChk/1
  Relational Operator2/1 -> Logical Operator/2
  Relational Operator1/1 -> Logical Operator/1
  VehPosChk_bsR0Info/1 -> Bus Selector1/1
  Bus Selector1/1 -> Right Front Conner Deviation Calculation (RFCDvtCalc)/2(RFCDvtCalc_lDvt)  "<R0_C0>"
  VehPosChk_bsL0Info/1 -> Bus Selector/1
  Bus Selector/1 -> Left Front Conner Deviation Calculation (LFCDvtCalc)/1(LFCDvtCalc_lDvt)  "<L0_C0>"
  VehPosChk_lAlrmLine_C/1 -> Relational Operator2/2, Relational Operator1/2
  Right Front Conner Deviation Calculation (RFCDvtCalc)/1(DvtCalc_lRgtDvt) -> Relational Operator2/1
  Left Front Conner Deviation Calculation (LFCDvtCalc)/1(DvtCalc_lLftDvt) -> Relational Operator1/1
  VehPosChk_DvtComp_C/1 -> Left Front Conner Deviation Calculation (LFCDvtCalc)/2(LFCDvtCalc_lDvtComp_C), Right Front Conner Deviation Calculation (RFCDvtCalc)/1(RFCDvtCalc_lDvtComp_C)

== system D53_LKAS_JLU_20200911_1116/LL/LLOn/LL State Determination (LLStateDet)/LL State Machine Conditions (LLSMCon)/Disable Condition (DisblC)/Lane Condition (LaneC)/Lane C1 Detection (LaneC1Det) ==
  LaneWDet_facmL0C1 : Inport
  LaneWDet_facmR0C1 : Inport  Port=2
  Abs : Abs
  Add : Sum  Inputs=+-  OutDataTypeStr=single
  Compare To Constant1 : simulink/Logic and Bit Operations/Compare To Constant  relop=>  const=0.040  OutDataTypeStr=boolean
  LaneC1Det_stLaneC1DetFlg : Outport
  wires:
  Abs/1 -> Compare To Constant1/1
  Compare To Constant1/1 -> LaneC1Det_stLaneC1DetFlg/1
  Add/1 -> Abs/1
  LaneWDet_facmL0C1/1 -> Add/1
  LaneWDet_facmR0C1/1 -> Add/2

== system D53_LKAS_JLU_20200911_1116/LL/LLOn/LL State Determination (LLStateDet)/LL State Machine Conditions (LLSMCon)/Disable Condition (DisblC)/Lane Condition (LaneC)/Lane Condition Synthesis (LaneCSyn) ==
  LaneCSyn_stLaneQlECFlg : Inport
  LaneCSyn_stLaneWDetFlg : Inport  Port=2
  LaneCSyn_stLaneCrvtDetFlg : Inport  Port=3
  LaneCSyn_stLaneC1DetFlg : Inport  Port=4
  Logical Operator3 : Logic  Operator=OR  Inputs=4  AllPortsSameDT=off  OutDataTypeStr=boolean
  LaneCSyn_stLaneCSyn : Outport
  wires:
  LaneCSyn_stLaneC1DetFlg/1 -> Logical Operator3/4
  LaneCSyn_stLaneWDetFlg/1 -> Logical Operator3/2
  Logical Operator3/1 -> LaneCSyn_stLaneCSyn/1
  LaneCSyn_stLaneCrvtDetFlg/1 -> Logical Operator3/3
  LaneCSyn_stLaneQlECFlg/1 -> Logical Operator3/1

== system D53_LKAS_JLU_20200911_1116/LL/LLOn/LL State Determination (LLStateDet)/LL State Machine Conditions (LLSMCon)/Disable Condition (DisblC)/Lane Condition (LaneC)/Lane Curvature Detection (LaneCrvtDet) ==
  LaneCrvtDet_crPrvwCrvt : Inport
  LaneCrvtDet_crLaneCrvtMax_C : Inport  Port=2
  Abs : Abs
  Constant : Constant  Value=0  OutDataTypeStr=single  SampleTime=-1
  Interval Test Dynamic : simulink/Logic and Bit Operations/Interval Test Dynamic  IntervalClosedRight=on  IntervalClosedLeft=on  OutDataTypeStr=boolean
      settings: SourceProductName=Simulink  SourceProductBaseCode=SL
  Logical Operator : Logic  Operator=NOT  AllPortsSameDT=off  OutDataTypeStr=boolean
  LaneCrvtDet_stLaneCrvtDetFlg : Outport
  wires:
  Abs/1 -> Interval Test Dynamic/2
  LaneCrvtDet_crPrvwCrvt/1 -> Abs/1
  Constant/1 -> Interval Test Dynamic/3
  LaneCrvtDet_crLaneCrvtMax_C/1 -> Interval Test Dynamic/1
  Logical Operator/1 -> LaneCrvtDet_stLaneCrvtDetFlg/1
  Interval Test Dynamic/1 -> Logical Operator/1

== system D53_LKAS_JLU_20200911_1116/LL/LLOn/LL State Determination (LLStateDet)/LL State Machine Conditions (LLSMCon)/Disable Condition (DisblC)/Lane Condition (LaneC)/Lane Quality Disable Condition (LaneQlDC) ==
  LaneQlDC_stFacmL0Ql : Inport
  LaneQlDC_stFacmR0Ql : Inport  Port=2
  Compare To Constant : simulink/Logic and Bit Operations/Compare To Constant  relop=<  const=3  OutDataTypeStr=boolean
  Compare To Constant1 : simulink/Logic and Bit Operations/Compare To Constant  relop=<  const=3  OutDataTypeStr=boolean
  Logical Operator : Logic  AllPortsSameDT=off  OutDataTypeStr=boolean
  LaneQlDC_stLaneQlDCFlg : Outport
  wires:
  Logical Operator/1 -> LaneQlDC_stLaneQlDCFlg/1
  Compare To Constant1/1 -> Logical Operator/2
  Compare To Constant/1 -> Logical Operator/1
  LaneQlDC_stFacmR0Ql/1 -> Compare To Constant1/1
  LaneQlDC_stFacmL0Ql/1 -> Compare To Constant/1

== system D53_LKAS_JLU_20200911_1116/LL/LLOn/LL State Determination (LLStateDet)/LL State Machine Conditions (LLSMCon)/Disable Condition (DisblC)/Lane Condition (LaneC)/Lane Width Detection (LaneWDet) ==
  LaneWDet_LaneWidth : Inport
  LaneWDet_lLaneWMax : Inport  Port=2
  LaneWDet_lLaneWMin : Inport  Port=3
  Abs1 : Abs
  Compare To Zero : simulink/Logic and Bit Operations/Compare To Zero  relop===  OutDataTypeStr=boolean
  Interval Test Dynamic : simulink/Logic and Bit Operations/Interval Test Dynamic  IntervalClosedRight=on  IntervalClosedLeft=on  OutDataTypeStr=boolean
      settings: SourceProductName=Simulink  SourceProductBaseCode=SL
  LaneWDet_stLaneWDetFlg : Outport
  wires:
  LaneWDet_LaneWidth/1 -> Abs1/1
  Abs1/1 -> Interval Test Dynamic/2
  LaneWDet_lLaneWMin/1 -> Interval Test Dynamic/3
  LaneWDet_lLaneWMax/1 -> Interval Test Dynamic/1
  Compare To Zero/1 -> LaneWDet_stLaneWDetFlg/1
  Interval Test Dynamic/1 -> Compare To Zero/1

== system D53_LKAS_JLU_20200911_1116/LL/LLOn/LL State Determination (LLStateDet)/LL State Machine Conditions (LLSMCon)/Disable Condition (DisblC)/Subsystem/Subsystem ==
  in1 : Inport
  Add : Sum
  Cast To Single : DataTypeConversion  OutDataTypeStr=uint8
  Memory : Memory  InheritSampleTime=on
  Saturation : Saturate  UpperLimit=1  LowerLimit=0
  Out1 : Outport
  wires:
  Saturation/1 -> Out1/1, Add/2
  Add/1 -> Memory/1
  Memory/1 -> Saturation/1
  in1/1 -> Cast To Single/1
  Cast To Single/1 -> Add/1

== system D53_LKAS_JLU_20200911_1116/LL/LLOn/LL State Determination (LLStateDet)/LL State Machine Conditions (LLSMCon)/Disable Condition (DisblC)/Subsystem/Subsystem1 ==
  in1 : Inport
  Add : Sum
  Cast To Single : DataTypeConversion  OutDataTypeStr=uint8
  Memory : Memory  InheritSampleTime=on
  Saturation : Saturate  UpperLimit=1  LowerLimit=0
  Out1 : Outport
  wires:
  Cast To Single/1 -> Add/1
  in1/1 -> Cast To Single/1
  Memory/1 -> Saturation/1
  Add/1 -> Memory/1
  Saturation/1 -> Add/2, Out1/1

== system D53_LKAS_JLU_20200911_1116/LL/LLOn/LL State Determination (LLStateDet)/LL State Machine Conditions (LLSMCon)/Disable Condition (DisblC)/Subsystem/Subsystem10 ==
  in1 : Inport
  Add : Sum
  Cast To Single : DataTypeConversion  OutDataTypeStr=uint8
  Memory : Memory  InheritSampleTime=on
  Saturation : Saturate  UpperLimit=1  LowerLimit=0
  Out1 : Outport
  wires:
  Saturation/1 -> Out1/1, Add/2
  Add/1 -> Memory/1
  Memory/1 -> Saturation/1
  in1/1 -> Cast To Single/1
  Cast To Single/1 -> Add/1

== system D53_LKAS_JLU_20200911_1116/LL/LLOn/LL State Determination (LLStateDet)/LL State Machine Conditions (LLSMCon)/Disable Condition (DisblC)/Subsystem/Subsystem11 ==
  in1 : Inport
  Add : Sum
  Cast To Single : DataTypeConversion  OutDataTypeStr=uint8
  Memory : Memory  InheritSampleTime=on
  Saturation : Saturate  UpperLimit=1  LowerLimit=0
  Out1 : Outport
  wires:
  Cast To Single/1 -> Add/1
  in1/1 -> Cast To Single/1
  Memory/1 -> Saturation/1
  Add/1 -> Memory/1
  Saturation/1 -> Add/2, Out1/1

== system D53_LKAS_JLU_20200911_1116/LL/LLOn/LL State Determination (LLStateDet)/LL State Machine Conditions (LLSMCon)/Disable Condition (DisblC)/Subsystem/Subsystem12 ==
  in1 : Inport
  Add : Sum
  Cast To Single : DataTypeConversion  OutDataTypeStr=uint8
  Memory : Memory  InheritSampleTime=on
  Saturation : Saturate  UpperLimit=1  LowerLimit=0
  Out1 : Outport
  wires:
  Saturation/1 -> Out1/1, Add/2
  Add/1 -> Memory/1
  Memory/1 -> Saturation/1
  in1/1 -> Cast To Single/1
  Cast To Single/1 -> Add/1

== system D53_LKAS_JLU_20200911_1116/LL/LLOn/LL State Determination (LLStateDet)/LL State Machine Conditions (LLSMCon)/Disable Condition (DisblC)/Subsystem/Subsystem13 ==
  in1 : Inport
  Add : Sum
  Cast To Single : DataTypeConversion  OutDataTypeStr=uint8
  Memory : Memory  InheritSampleTime=on
  Saturation : Saturate  UpperLimit=1  LowerLimit=0
  Out1 : Outport
  wires:
  Cast To Single/1 -> Add/1
  in1/1 -> Cast To Single/1
  Memory/1 -> Saturation/1
  Add/1 -> Memory/1
  Saturation/1 -> Add/2, Out1/1

== system D53_LKAS_JLU_20200911_1116/LL/LLOn/LL State Determination (LLStateDet)/LL State Machine Conditions (LLSMCon)/Disable Condition (DisblC)/Subsystem/Subsystem14 ==
  in1 : Inport
  Add : Sum
  Cast To Single : DataTypeConversion  OutDataTypeStr=uint8
  Memory : Memory  InheritSampleTime=on
  Saturation : Saturate  UpperLimit=1  LowerLimit=0
  Out1 : Outport
  wires:
  Cast To Single/1 -> Add/1
  in1/1 -> Cast To Single/1
  Memory/1 -> Saturation/1
  Add/1 -> Memory/1
  Saturation/1 -> Add/2, Out1/1

== system D53_LKAS_JLU_20200911_1116/LL/LLOn/LL State Determination (LLStateDet)/LL State Machine Conditions (LLSMCon)/Disable Condition (DisblC)/Subsystem/Subsystem15 ==
  in1 : Inport
  Add : Sum
  Cast To Single : DataTypeConversion  OutDataTypeStr=uint8
  Memory : Memory  InheritSampleTime=on
  Saturation : Saturate  UpperLimit=1  LowerLimit=0
  Out1 : Outport
  wires:
  Saturation/1 -> Out1/1, Add/2
  Add/1 -> Memory/1
  Memory/1 -> Saturation/1
  in1/1 -> Cast To Single/1
  Cast To Single/1 -> Add/1

== system D53_LKAS_JLU_20200911_1116/LL/LLOn/LL State Determination (LLStateDet)/LL State Machine Conditions (LLSMCon)/Disable Condition (DisblC)/Subsystem/Subsystem16 ==
  in1 : Inport
  Add : Sum
  Cast To Single : DataTypeConversion  OutDataTypeStr=uint8
  Memory : Memory  InheritSampleTime=on
  Saturation : Saturate  UpperLimit=1  LowerLimit=0
  Out1 : Outport
  wires:
  Saturation/1 -> Out1/1, Add/2
  Add/1 -> Memory/1
  Memory/1 -> Saturation/1
  in1/1 -> Cast To Single/1
  Cast To Single/1 -> Add/1

== system D53_LKAS_JLU_20200911_1116/LL/LLOn/LL State Determination (LLStateDet)/LL State Machine Conditions (LLSMCon)/Disable Condition (DisblC)/Subsystem/Subsystem17 ==
  in1 : Inport
  Add : Sum
  Cast To Single : DataTypeConversion  OutDataTypeStr=uint8
  Memory : Memory  InheritSampleTime=on
  Saturation : Saturate  UpperLimit=1  LowerLimit=0
  Out1 : Outport
  wires:
  Cast To Single/1 -> Add/1
  in1/1 -> Cast To Single/1
  Memory/1 -> Saturation/1
  Add/1 -> Memory/1
  Saturation/1 -> Add/2, Out1/1

== system D53_LKAS_JLU_20200911_1116/LL/LLOn/LL State Determination (LLStateDet)/LL State Machine Conditions (LLSMCon)/Disable Condition (DisblC)/Subsystem/Subsystem2 ==
  in1 : Inport
  Add : Sum
  Cast To Single : DataTypeConversion  OutDataTypeStr=uint8
  Memory : Memory  InheritSampleTime=on
  Saturation : Saturate  UpperLimit=1  LowerLimit=0
  Out1 : Outport
  wires:
  Cast To Single/1 -> Add/1
  in1/1 -> Cast To Single/1
  Memory/1 -> Saturation/1
  Add/1 -> Memory/1
  Saturation/1 -> Add/2, Out1/1

== system D53_LKAS_JLU_20200911_1116/LL/LLOn/LL State Determination (LLStateDet)/LL State Machine Conditions (LLSMCon)/Disable Condition (DisblC)/Subsystem/Subsystem3 ==
  in1 : Inport
  Add : Sum
  Cast To Single : DataTypeConversion  OutDataTypeStr=uint8
  Memory : Memory  InheritSampleTime=on
  Saturation : Saturate  UpperLimit=1  LowerLimit=0
  Out1 : Outport
  wires:
  Saturation/1 -> Out1/1, Add/2
  Add/1 -> Memory/1
  Memory/1 -> Saturation/1
  in1/1 -> Cast To Single/1
  Cast To Single/1 -> Add/1

== system D53_LKAS_JLU_20200911_1116/LL/LLOn/LL State Determination (LLStateDet)/LL State Machine Conditions (LLSMCon)/Disable Condition (DisblC)/Subsystem/Subsystem4 ==
  in1 : Inport
  Add : Sum
  Cast To Single : DataTypeConversion  OutDataTypeStr=uint8
  Memory : Memory  InheritSampleTime=on
  Saturation : Saturate  UpperLimit=1  LowerLimit=0
  Out1 : Outport
  wires:
  Cast To Single/1 -> Add/1
  in1/1 -> Cast To Single/1
  Memory/1 -> Saturation/1
  Add/1 -> Memory/1
  Saturation/1 -> Add/2, Out1/1

== system D53_LKAS_JLU_20200911_1116/LL/LLOn/LL State Determination (LLStateDet)/LL State Machine Conditions (LLSMCon)/Disable Condition (DisblC)/Subsystem/Subsystem5 ==
  in1 : Inport
  Add : Sum
  Cast To Single : DataTypeConversion  OutDataTypeStr=uint8
  Memory : Memory  InheritSampleTime=on
  Saturation : Saturate  UpperLimit=1  LowerLimit=0
  Out1 : Outport
  wires:
  Saturation/1 -> Out1/1, Add/2
  Add/1 -> Memory/1
  Memory/1 -> Saturation/1
  in1/1 -> Cast To Single/1
  Cast To Single/1 -> Add/1
